simulink model "main"  (Simulink 7.3)
settings: Solver=ode3  StartTime=0.0  StopTime=inf  FixedStep=0.01  RelTol=1e-3
undefined symbols (not defined in the file or in its folder): serial
libraries: simulink x9, NAV420Lib x3, NAV420DecodeLib x3, NAV420ExLib x3, instrumentlib x3
settings Model: Creator=djulzz  LastModifiedBy=Administrateur

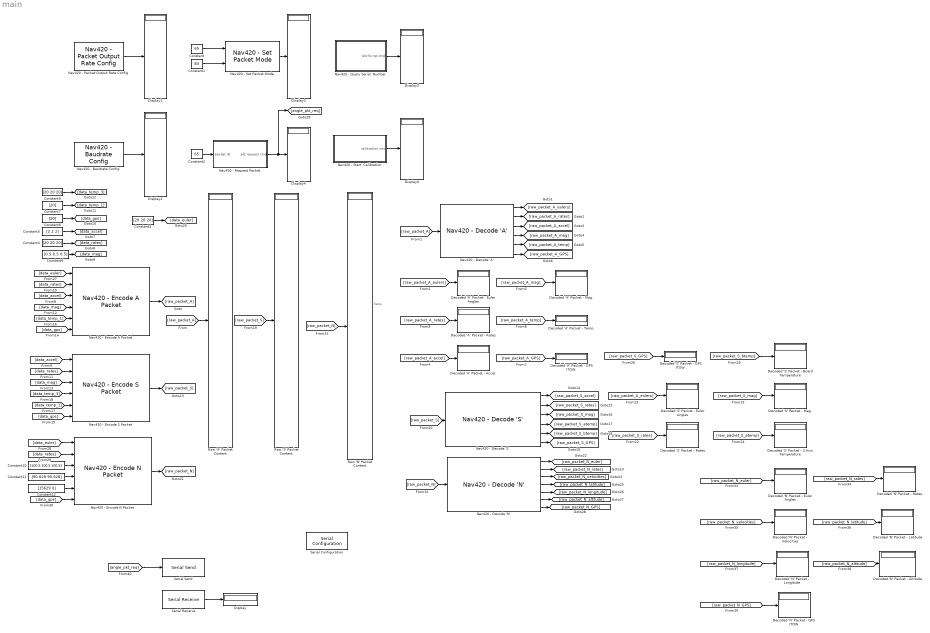
== system main ==
  note: here
  Constant : Constant  Value=65  OutDataTypeMode=int8  OutDataType=fixdt(1, 16)  OutScaling=2^0  OutDataTypeStr=int8  SampleTime=-1
  Constant1 : Constant  Value=83  OutDataTypeMode=int8  OutDataType=fixdt(1, 16)  OutScaling=2^0  OutDataTypeStr=int8  SampleTime=-1
  Constant10 : Constant  Value=[100.5 100.5 100.5]  OutDataTypeMode=double  OutDataType=fixdt(1, 16)  OutScaling=2^0  OutDataTypeStr=double  SampleTime=-1
  Constant11 : Constant  Value=[90.628 90.628]  OutDataTypeMode=double  OutDataType=fixdt(1, 16)  OutScaling=2^0  OutDataTypeStr=double  SampleTime=-1
  Constant12 : Constant  Value=[15629.0]  OutDataTypeMode=double  OutDataType=fixdt(1, 16)  OutScaling=2^0  OutDataTypeStr=double  SampleTime=-1
  Constant2 : Constant  Value=65  OutDataTypeMode=int8  OutDataType=fixdt(1, 16)  OutScaling=2^0  OutDataTypeStr=int8  SampleTime=-1
  Constant3 : Constant  Value=[20 20 20]  OutDataTypeMode=double  OutDataType=fixdt(1, 16)  OutScaling=2^0  OutDataTypeStr=double  SampleTime=-1
  Constant4 : Constant  Value=[20 20 20]  OutDataTypeMode=double  OutDataType=fixdt(1, 16)  OutScaling=2^0  OutDataTypeStr=double  SampleTime=-1
  Constant5 : Constant  Value=[2 2 2]  OutDataTypeMode=double  OutDataType=fixdt(1, 16)  OutScaling=2^0  OutDataTypeStr=double  SampleTime=-1
  Constant6 : Constant  Value=[0.5 0.5 0.5]  OutDataTypeMode=double  OutDataType=fixdt(1, 16)  OutScaling=2^0  OutDataTypeStr=double  SampleTime=-1
  Constant7 : Constant  Value=[20]  OutDataTypeMode=double  OutDataType=fixdt(1, 16)  OutScaling=2^0  OutDataTypeStr=double  SampleTime=-1
  Constant8 : Constant  Value=[20]  OutDataTypeMode=uint16  OutDataType=fixdt(1, 16)  OutScaling=2^0  OutDataTypeStr=uint16  SampleTime=-1
  Constant9 : Constant  Value=[20 20 20]  OutDataTypeMode=double  OutDataType=fixdt(1, 16)  OutScaling=2^0  OutDataTypeStr=double  SampleTime=-1
  Decoded 'A' Packet - Accel. : Display
  Decoded 'A' Packet - Euler Angles : Display
  Decoded 'A' Packet - GPS ITOW. : Display
  Decoded 'A' Packet - Mag. : Display
  Decoded 'A' Packet - Rates : Display
  Decoded 'A' Packet - Temp. : Display
  Decoded 'N' Packet - Altitude : Display
  Decoded 'N' Packet - Euler Angles : Display
  Decoded 'N' Packet - GPS ITOW : Display
  Decoded 'N' Packet - Latitude : Display
  Decoded 'N' Packet - Longitude : Display
  Decoded 'N' Packet - Rates : Display
  Decoded 'N' Packet - Velocities : Display
  Decoded 'S' Packet - 3 Axis Temperature : Display
  Decoded 'S' Packet - Board Temperature : Display
  Decoded 'S' Packet - Euler Angles : Display
  Decoded 'S' Packet - GPS ITOW. : Display
  Decoded 'S' Packet - Mag. : Display
  Decoded 'S' Packet - Rates : Display
  Display{,1..6} (7 alike) : Display
      settings: Format=hex (Stored Integer)
  Nav420 - Baudrate Config : NAV420Lib/Nav420 - Baudrate Config  SystemSampleTime=-1  baudrateIndex=9600  SaveConfig=off
  Nav420 - Decode 'A' : NAV420DecodeLib/Nav420 - Decode 'A'  SystemSampleTime=-1
  Nav420 - Decode 'N' : NAV420DecodeLib/Nav420 - Decode 'N'  SystemSampleTime=-1
  Nav420 - Decode 'S' : NAV420DecodeLib/Nav420 - Decode 'S'  SystemSampleTime=-1
  Nav420 - Encode A Packet : NAV420ExLib/Nav420 - Encode A Packet  SystemSampleTime=-1
  Nav420 - Encode N Packet : NAV420ExLib/Nav420 - Encode N Packet  SystemSampleTime=-1
  Nav420 - Encode S Packet : NAV420ExLib/Nav420 - Encode S Packet  SystemSampleTime=-1
  Nav420 - Packet Output Rate Config : NAV420Lib/Nav420 - Packet Output Rate Config  SystemSampleTime=-1  shouldSave=off  output_rate=100
  Nav420 - Query Serial  Number : Subsystem  AncestorBlock="NAV420Lib/Nav420 - Query Serial  Number"
  Nav420 - Request Packet : Subsystem  AncestorBlock=NAV420Lib/Nav420 - Request Packet
  Nav420 - Set Packet Mode : NAV420Lib/Nav420 - Set Packet Mode  SystemSampleTime=-1
      link override From4: GotoTag=Set
      link override Goto4: GotoTag=Set
  Nav420 - Start  Calibration : Subsystem  AncestorBlock="NAV420Lib/Nav420 - Start  Calibration"
  Raw 'A' Packet Content : Display
      settings: Format=hex (Stored Integer)
  Raw 'N' Packet Content : Display
      settings: Format=hex (Stored Integer)
  Raw 'S' Packet Content : Display
      settings: Format=hex (Stored Integer)
  Serial Configuration : instrumentlib/Serial Configuration  Priority=-200000  DialogController=instrumentcreatedialog  DialogControllerArgs=DataTag0  ComPortMenu=COM4  ComPort=COM4  ObjConstructor=serial('COM4');  BaudRate=38400  DataBits=8  Parity=none  StopBits=1  FlowControl=none  Timeout=10  ByteOrder=LittleEndian
  Serial Receive : instrumentlib/Serial Receive  DialogController=instrumentcreatedialog  DialogControllerArgs=DataTag1  ComPortMenu=COM4  ComPort=COM4  ObjConstructor=serial('COM4');  Terminator=<none>  DataSize="[1  35]"  DataType=uint8  EnableBlockingMode=on  ActionDataUnavailable=Output last received value  CustomValue=0  SampleTime=-1
  Serial Send : instrumentlib/Serial Send  DialogController=instrumentcreatedialog  DialogControllerArgs=DataTag2  ComPortMenu=COM4  ComPort=COM4  Terminator=<none>  EnableBlockingMode=on
  wires:
  Nav420 - Packet Output Rate Config/1 -> Display1/1
  Nav420 - Baudrate Config/1 -> Display2/1
  Constant1/1 -> Nav420 - Set Packet Mode/2
  Constant/1 -> Nav420 - Set Packet Mode/1
  Nav420 - Set Packet Mode/1 -> Display3/1
  Constant2/1 -> Nav420 - Request Packet/1(packet ID)
  Nav420 - Request Packet/1(pkt request cmd) -> Display4/1, [angle_pkt_req]
  Nav420 - Query Serial  Number/1(pkt fw rqt cmd) -> Display5/1
  Nav420 - Start  Calibration/1(calibration cmd) -> Display6/1
  Nav420 - Encode A Packet/1 -> [raw_packet_A]
  [raw_packet_A] -> Raw 'A' Packet Content/1
  Nav420 - Decode 'A'/1 -> [raw_packet_A_eulers]
  Nav420 - Decode 'A'/2 -> [raw_packet_A_rates]
  Nav420 - Decode 'A'/3 -> [raw_packet_A_accel]
  Nav420 - Decode 'A'/4 -> [raw_packet_A_mag]
  Nav420 - Decode 'A'/5 -> [raw_packet_A_temp]
  Nav420 - Decode 'A'/6 -> [raw_packet_A_GPS]
  [raw_packet_A_eulers] -> Decoded 'A' Packet - Euler Angles/1
  [raw_packet_A_rates] -> Decoded 'A' Packet - Rates/1
  [raw_packet_A_accel] -> Decoded 'A' Packet - Accel./1
  [raw_packet_A_mag] -> Decoded 'A' Packet - Mag./1
  [raw_packet_A_temp] -> Decoded 'A' Packet - Temp./1
  [raw_packet_A_GPS] -> Decoded 'A' Packet - GPS ITOW./1
  [raw_packet_A] -> Nav420 - Decode 'A'/1
  Constant5/1 -> [data_accel]
  [data_accel] -> Nav420 - Encode A Packet/3
  [data_accel] -> Nav420 - Encode S Packet/1
  Constant4/1 -> [data_rates]
  [data_rates] -> Nav420 - Encode A Packet/2
  [data_rates] -> Nav420 - Encode S Packet/2
  Constant6/1 -> [data_mag]
  [data_mag] -> Nav420 - Encode A Packet/4
  [data_mag] -> Nav420 - Encode S Packet/3
  Constant8/1 -> [data_gps]
  [data_gps] -> Nav420 - Encode A Packet/6
  [data_gps] -> Nav420 - Encode S Packet/6
  Constant7/1 -> [data_temp_1]
  [data_temp_1] -> Nav420 - Encode A Packet/5
  [data_temp_1] -> Nav420 - Encode S Packet/5
  Constant9/1 -> [data_temp_3]
  [data_temp_3] -> Nav420 - Encode S Packet/4
  [raw_packet_S] -> Raw 'S' Packet Content/1
  [raw_packet_S] -> Nav420 - Decode 'S'/1
  Nav420 - Decode 'S'/1 -> [raw_packet_S_accel]
  Nav420 - Decode 'S'/2 -> [raw_packet_S_rates]
  Nav420 - Decode 'S'/3 -> [raw_packet_S_mag]
  Nav420 - Decode 'S'/4 -> [raw_packet_S_atemp]
  Nav420 - Decode 'S'/5 -> [raw_packet_S_btemp]
  Nav420 - Decode 'S'/6 -> [raw_packet_S_GPS]
  [raw_packet_A_eulers] -> Decoded 'S' Packet - Euler Angles/1
  [raw_packet_S_rates] -> Decoded 'S' Packet - Rates/1
  [raw_packet_S_mag] -> Decoded 'S' Packet - Mag./1
  [raw_packet_S_atemp] -> Decoded 'S' Packet - 3 Axis Temperature/1
  [raw_packet_S_btemp] -> Decoded 'S' Packet - Board Temperature/1
  [raw_packet_S_GPS] -> Decoded 'S' Packet - GPS ITOW./1
  Nav420 - Encode S Packet/1 -> [raw_packet_S]
  Constant3/1 -> [data_euler]
  [data_euler] -> Nav420 - Encode A Packet/1
  [data_euler] -> Nav420 - Encode N Packet/1
  [data_rates] -> Nav420 - Encode N Packet/2
  Constant10/1 -> Nav420 - Encode N Packet/3
  Constant11/1 -> Nav420 - Encode N Packet/4
  Constant12/1 -> Nav420 - Encode N Packet/5
  [data_gps] -> Nav420 - Encode N Packet/6
  [raw_packet_N] -> Raw 'N' Packet Content/1
  [raw_packet_N] -> Nav420 - Decode 'N'/1
  Nav420 - Decode 'N'/7 -> [raw_packet_N_GPS]
  Nav420 - Decode 'N'/6 -> [raw_packet_N_altitude]
  Nav420 - Decode 'N'/5 -> [raw_packet_N_longitude]
  Nav420 - Decode 'N'/4 -> [raw_packet_N_latitude]
  Nav420 - Decode 'N'/3 -> [raw_packet_N_velocities]
  Nav420 - Decode 'N'/2 -> [raw_packet_N_rates]
  Nav420 - Decode 'N'/1 -> [raw_packet_N_euler]
  [raw_packet_N_euler] -> Decoded 'N' Packet - Euler Angles/1
  [raw_packet_N_rates] -> Decoded 'N' Packet - Rates/1
  [raw_packet_N_velocities] -> Decoded 'N' Packet - Velocities/1
  [raw_packet_N_latitude] -> Decoded 'N' Packet - Latitude/1
  [raw_packet_N_longitude] -> Decoded 'N' Packet - Longitude/1
  [raw_packet_N_altitude] -> Decoded 'N' Packet - Altitude/1
  [raw_packet_N_GPS] -> Decoded 'N' Packet - GPS ITOW/1
  Nav420 - Encode N Packet/1 -> [raw_packet_N]
  [angle_pkt_req] -> Serial Send/1
  Serial Receive/1 -> Display/1

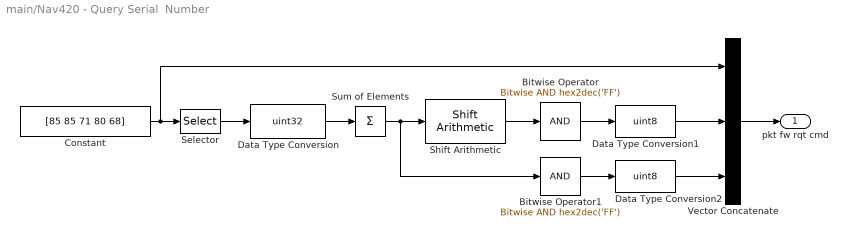
== system main/Nav420 - Query Serial  Number ==
  Bitwise Operator : simulink/Logic and Bit Operations/Bitwise Operator  logicop=AND  UseBitMask=on  BitMask=hex2dec('FF')  BitMaskRealWorld=Stored Integer
  Bitwise Operator1 : simulink/Logic and Bit Operations/Bitwise Operator  logicop=AND  UseBitMask=on  BitMask=hex2dec('FF')  BitMaskRealWorld=Stored Integer
  Constant : Constant  Value=[85 85 71 80 68]  OutDataTypeMode=uint8  OutDataType=fixdt(1, 16)  OutScaling=2^0  OutDataTypeStr=uint8
  Data Type Conversion : DataTypeConversion  OutDataTypeMode=uint32  OutDataType=fixdt(1, 16)  OutScaling=2^0  OutDataTypeStr=uint32
  Data Type Conversion1 : DataTypeConversion  OutDataTypeMode=uint8  OutDataType=fixdt(1, 16)  OutScaling=2^0  OutDataTypeStr=uint8
  Data Type Conversion2 : DataTypeConversion  OutDataTypeMode=uint8  OutDataType=fixdt(1, 16)  OutScaling=2^0  OutDataTypeStr=uint8
  Selector : Selector  InputPortWidth=5  IndexOptions=Index vector (dialog)  Indices=[3 4 5]  OutputSizes=1
  Shift Arithmetic : simulink/Logic and Bit Operations/Shift Arithmetic  SystemSampleTime=-1  nBitShiftRight=8  nBinPtShiftRight=0
  Sum of Elements : Sum  Inputs=+  OutDataType=fixdt(1, 16)  OutScaling=2^-10
  Vector Concatenate : Concatenate  NumInputs=3  Mode=Vector
  pkt fw rqt cmd : Outport  OutDataType=fixdt(1, 16)  OutScaling=2^0
  wires:
  Vector Concatenate/1 -> pkt fw rqt cmd/1
  Data Type Conversion1/1 -> Vector Concatenate/2
  Data Type Conversion2/1 -> Vector Concatenate/3
  Bitwise Operator1/1 -> Data Type Conversion2/1
  Bitwise Operator/1 -> Data Type Conversion1/1
  Shift Arithmetic/1 -> Bitwise Operator/1
  Sum of Elements/1 -> Bitwise Operator1/1, Shift Arithmetic/1
  Data Type Conversion/1 -> Sum of Elements/1
  Selector/1 -> Data Type Conversion/1
  Constant/1 -> Selector/1, Vector Concatenate/1

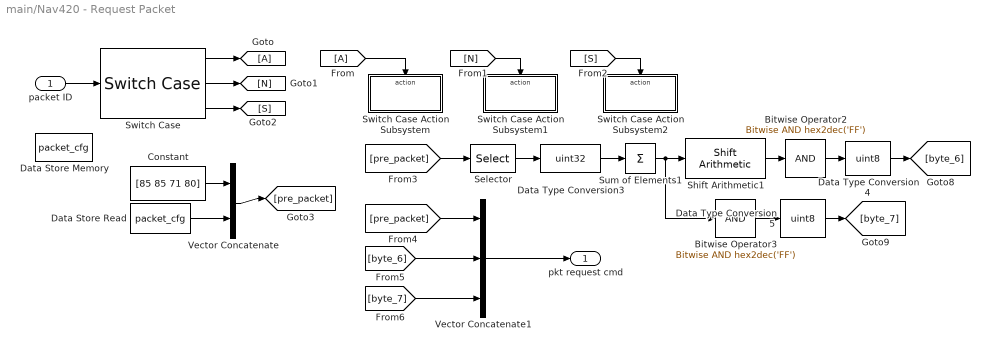
== system main/Nav420 - Request Packet ==
  packet ID : Inport  DataType=int8  OutDataType=fixdt(1, 16)  OutScaling=2^0  OutDataTypeStr=int8
  Bitwise Operator2 : simulink/Logic and Bit Operations/Bitwise Operator  logicop=AND  UseBitMask=on  BitMask=hex2dec('FF')  BitMaskRealWorld=Stored Integer
  Bitwise Operator3 : simulink/Logic and Bit Operations/Bitwise Operator  logicop=AND  UseBitMask=on  BitMask=hex2dec('FF')  BitMaskRealWorld=Stored Integer
  Constant : Constant  Value=[85 85 71 80]  OutDataTypeMode=uint8  OutDataType=fixdt(1, 16)  OutScaling=2^0  OutDataTypeStr=uint8  SampleTime=-1
  Data Store Memory : DataStoreMemory  DataStoreName=packet_cfg  DataType=uint8  OutDataType=fixdt(1, 16)  OutScaling=2^0  OutDataTypeStr=uint8
  Data Store Read : DataStoreRead  DataStoreName=packet_cfg  SampleTime=0
  Data Type Conversion3 : DataTypeConversion  OutDataTypeMode=uint32  OutDataType=fixdt(1, 16)  OutScaling=2^0  OutDataTypeStr=uint32  RndMeth=Nearest
  Data Type Conversion4 : DataTypeConversion  OutDataTypeMode=uint8  OutDataType=fixdt(1, 16)  OutScaling=2^0  OutDataTypeStr=uint8  RndMeth=Nearest
  Data Type Conversion5 : DataTypeConversion  OutDataTypeMode=uint8  OutDataType=fixdt(1, 16)  OutScaling=2^0  OutDataTypeStr=uint8  RndMeth=Nearest
  Selector : Selector  InputPortWidth=5  IndexOptions=Index vector (dialog)  Indices=[3 4 5]  OutputSizes=1
  Shift Arithmetic1 : simulink/Logic and Bit Operations/Shift Arithmetic  SystemSampleTime=-1  nBitShiftRight=8  nBinPtShiftRight=0
  Sum of Elements1 : Sum  Inputs=+  OutDataType=fixdt(1, 16)  OutScaling=2^-10
  Switch Case : SwitchCase  CaseConditions={65,78}
  Switch Case Action Subsystem : Subsystem  TreatAsAtomicUnit=on
  Switch Case Action Subsystem1 : Subsystem  TreatAsAtomicUnit=on
  Switch Case Action Subsystem2 : Subsystem  TreatAsAtomicUnit=on
  Vector Concatenate : Concatenate  Mode=Vector
  Vector Concatenate1 : Concatenate  NumInputs=3  Mode=Vector
  pkt request cmd : Outport  DataType=uint8  OutDataType=fixdt(1, 16)  OutScaling=2^0  OutDataTypeStr=uint8
  wires:
  Vector Concatenate1/1 -> pkt request cmd/1
  [byte_7] -> Vector Concatenate1/3
  [byte_6] -> Vector Concatenate1/2
  [pre_packet] -> Vector Concatenate1/1
  Data Type Conversion3/1 -> Sum of Elements1/1
  Sum of Elements1/1 -> Bitwise Operator3/1, Shift Arithmetic1/1
  Data Type Conversion5/1 -> [byte_7]
  Data Type Conversion4/1 -> [byte_6]
  Bitwise Operator3/1 -> Data Type Conversion5/1
  Bitwise Operator2/1 -> Data Type Conversion4/1
  Shift Arithmetic1/1 -> Bitwise Operator2/1
  Selector/1 -> Data Type Conversion3/1
  [pre_packet] -> Selector/1
  Vector Concatenate/1 -> [pre_packet]
  Data Store Read/1 -> Vector Concatenate/2
  Constant/1 -> Vector Concatenate/1
  [S] -> Switch Case Action Subsystem2/Action
  [N] -> Switch Case Action Subsystem1/Action
  [A] -> Switch Case Action Subsystem/Action
  Switch Case/3 -> [S]
  Switch Case/2 -> [N]
  Switch Case/1 -> [A]
  packet ID/1 -> Switch Case/1

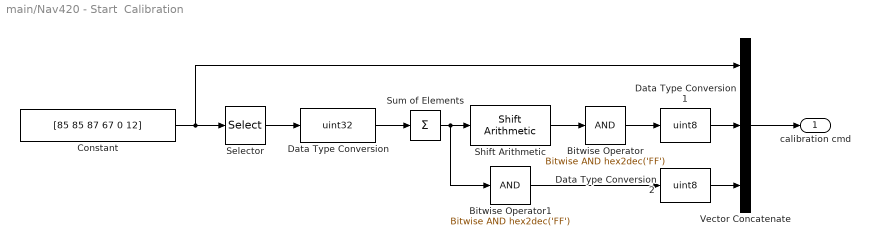
== system main/Nav420 - Start  Calibration ==
  Bitwise Operator : simulink/Logic and Bit Operations/Bitwise Operator  logicop=AND  UseBitMask=on  BitMask=hex2dec('FF')  BitMaskRealWorld=Stored Integer
  Bitwise Operator1 : simulink/Logic and Bit Operations/Bitwise Operator  logicop=AND  UseBitMask=on  BitMask=hex2dec('FF')  BitMaskRealWorld=Stored Integer
  Constant : Constant  Value=[85 85 87 67 0 12]  OutDataTypeMode=uint8  OutDataType=fixdt(1, 16)  OutScaling=2^0  OutDataTypeStr=uint8  SampleTime=-1
  Data Type Conversion : DataTypeConversion  OutDataTypeMode=uint32  OutDataType=fixdt(1, 16)  OutScaling=2^0  OutDataTypeStr=uint32
  Data Type Conversion1 : DataTypeConversion  OutDataTypeMode=uint8  OutDataType=fixdt(1, 16)  OutScaling=2^0  OutDataTypeStr=uint8
  Data Type Conversion2 : DataTypeConversion  OutDataTypeMode=uint8  OutDataType=fixdt(1, 16)  OutScaling=2^0  OutDataTypeStr=uint8
  Selector : Selector  InputPortWidth=6  IndexOptions=Index vector (dialog)  Indices=[3 4 5 6]  OutputSizes=1
  Shift Arithmetic : simulink/Logic and Bit Operations/Shift Arithmetic  SystemSampleTime=-1  nBitShiftRight=8  nBinPtShiftRight=0
  Sum of Elements : Sum  Inputs=+  OutDataType=fixdt(1, 16)  OutScaling=2^-10
  Vector Concatenate : Concatenate  NumInputs=3  Mode=Vector
  calibration cmd : Outport  DataType=uint8  OutDataType=fixdt(1, 16)  OutScaling=2^0  OutDataTypeStr=uint8
  wires:
  Vector Concatenate/1 -> calibration cmd/1
  Data Type Conversion1/1 -> Vector Concatenate/2
  Data Type Conversion2/1 -> Vector Concatenate/3
  Bitwise Operator1/1 -> Data Type Conversion2/1
  Bitwise Operator/1 -> Data Type Conversion1/1
  Shift Arithmetic/1 -> Bitwise Operator/1
  Sum of Elements/1 -> Bitwise Operator1/1, Shift Arithmetic/1
  Data Type Conversion/1 -> Sum of Elements/1
  Selector/1 -> Data Type Conversion/1
  Constant/1 -> Selector/1, Vector Concatenate/1

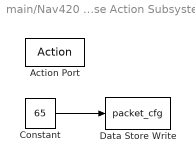
== system main/Nav420 - Request Packet/Switch Case Action Subsystem ==
  Action Port : ActionPort  ActionType=case
  Constant : Constant  Value=65  OutDataTypeMode=uint8  OutDataType=fixdt(1, 16)  OutScaling=2^0  OutDataTypeStr=uint8  SampleTime=-1
  Data Store Write : DataStoreWrite  DataStoreName=packet_cfg  SampleTime=-1
  wires:
  Constant/1 -> Data Store Write/1

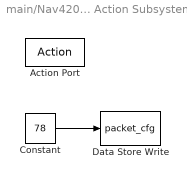
== system main/Nav420 - Request Packet/Switch Case Action Subsystem1 ==
  Action Port : ActionPort  ActionType=case
  Constant : Constant  Value=78  OutDataTypeMode=uint8  OutDataType=fixdt(1, 16)  OutScaling=2^0  OutDataTypeStr=uint8  SampleTime=-1
  Data Store Write : DataStoreWrite  DataStoreName=packet_cfg  SampleTime=-1
  wires:
  Constant/1 -> Data Store Write/1

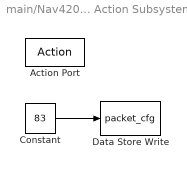
== system main/Nav420 - Request Packet/Switch Case Action Subsystem2 ==
  Action Port : ActionPort  ActionType=default
  Constant : Constant  Value=83  OutDataTypeMode=uint8  OutDataType=fixdt(1, 16)  OutScaling=2^0  OutDataTypeStr=uint8  SampleTime=-1
  Data Store Write : DataStoreWrite  DataStoreName=packet_cfg  SampleTime=-1
  wires:
  Constant/1 -> Data Store Write/1
